simulink model "model3"  (R2023a)
settings: Solver=FixedStepAuto  StartTime=0.0  StopTime=50.0  FixedStep=0.0001  RelTol=1e-3
settings Model: Creator=evdokiiagalkina  LastModifiedBy=evdokiiagalkina

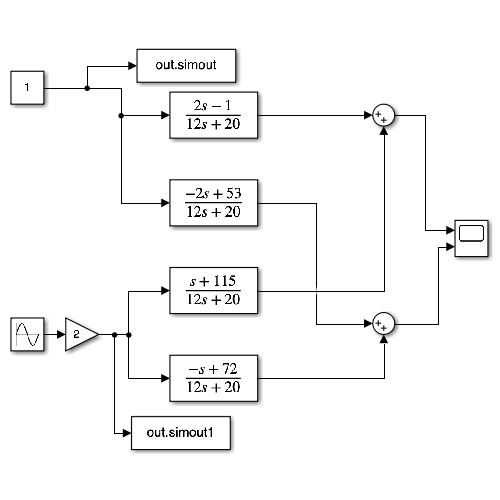
[thumbnail: Simulink's stored preview of the top-level diagram]
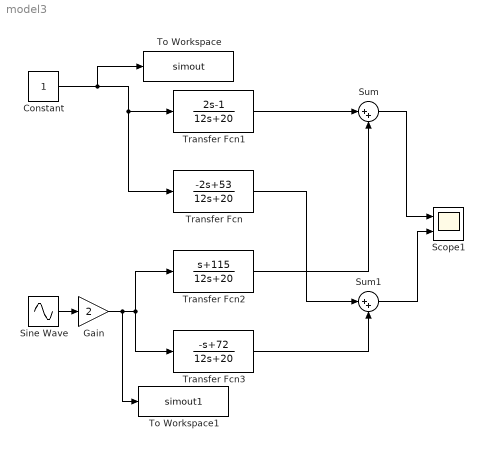
== system model3 ==
  Constant : Constant  SampleTime=-1
  Gain : Gain  Gain=2
  Scope1 : Scope  NumInputPorts=2
  Sine Wave : Sin  SampleTime=0
  Sum : Sum  Inputs=|++
  Sum1 : Sum  Inputs=|++
  To Workspace : ToWorkspace  VariableName=simout  SaveFormat=Timeseries  SampleTime=-1
  To Workspace1 : ToWorkspace  VariableName=simout1  SaveFormat=Timeseries  SampleTime=-1
  Transfer Fcn : TransferFcn  Numerator=[-2 53]  Denominator=[12 20]
  Transfer Fcn1 : TransferFcn  Numerator=[2 -1]  Denominator=[12 20]
  Transfer Fcn2 : TransferFcn  Numerator=[1 115]  Denominator=[12 20]
  Transfer Fcn3 : TransferFcn  Numerator=[-1 72]  Denominator=[12 20]
  wires:
  Sine Wave/1 -> Gain/1
  Transfer Fcn1/1 -> Sum/1
  Transfer Fcn2/1 -> Sum/2
  Transfer Fcn/1 -> Sum1/1
  Transfer Fcn3/1 -> Sum1/2
  Sum/1 -> Scope1/1
  Sum1/1 -> Scope1/2
  Constant/1 -> To Workspace/1, Transfer Fcn/1, Transfer Fcn1/1
  Gain/1 -> To Workspace1/1, Transfer Fcn3/1, Transfer Fcn2/1
